simulink model "sim_pendulum"  (R2025b)
settings: Solver=FixedStepAuto  StartTime=0.0  StopTime=30  FixedStep=0.02  RelTol=1e-6
values from neighbouring files (symbols this model uses):
  c1 = m1*L_2 + m2 * LR    (= 0.0141005)    [sim_main.m]
  c2 = m1*L2_4 + m2 * LR2    (= 0.001480019375)    [sim_main.m]
  dx0 = 0    [KF_EKF_SIM_TEST.m]    (also in sim_main.m)
  g = 9.81    [sim_main.m]
  m1 = 0.0540    (= 0.054)    [sim_main.m]
  m2 = 0.0965    [sim_main.m]
  mu = 0.00015    [sim_main.m]
  x0 = [x0;dx0]    [KF_EKF_SIM_TEST.m]    (also in nss_pendulum_sim.m = zeros(2 + w_disturbance, 1); nss_pendulum_sim_dynamicchar.m = zeros(n, 1); nss_pendulum_sim_staticchar.m = zeros(n, 1); sim_main.m = deg2rad(45))
  xi = 0.0003    [sim_main.m]
libraries: simulink_extras x1
settings Model: Creator=rjrad  LastModifiedBy=rjrad
settings DataIOCC: SaveOutput=off  DSMLogging=off  SaveTime=off  ReturnWorkspaceOutputs=off

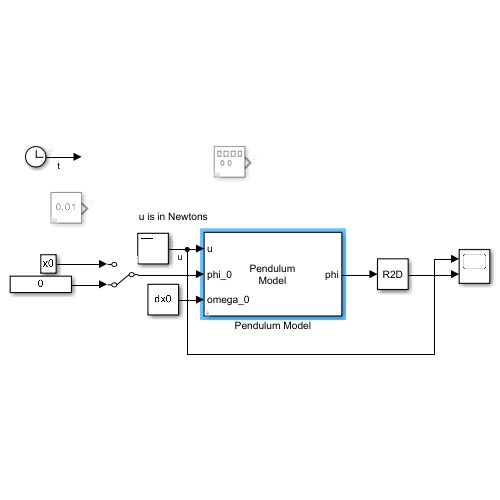
[thumbnail: Simulink's stored preview of the top-level diagram]
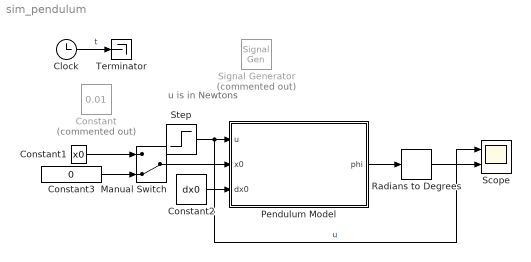
== system sim_pendulum ==
  note: u is in Newtons
  Clock : Clock
  Constant : Constant  Commented=on  Value=0.01
  Constant1 : Constant  Value=x0
  Constant2 : Constant  Value=dx0
  Constant3 : Constant  Value=0
  Manual Switch : ManualSwitch  CurrentSetting=0
  Pendulum Model : Subsystem  mask{g=g, b=xi, c1=c1, c2=c2}
      mask prompts: g "Gravitational acceleration"; b "Damping coefficient"; c1 "Inertia 1"; c2 "Inertia 2"
      mask Display:
      | disp('Pendulum\nModel');
      | port_label('output', 1, 'phi');
      | port_label('input', 1, 'u');
      | port_label('input', 2, 'phi_0');
      | port_label('input', 3, 'omega_0');
  Radians to Degrees : simulink_extras/Transformations/Radians to Degrees
  Scope : Scope  NumInputPorts=2
      settings: ActiveDisplayYMinimum=-15.510014538486551  ActiveDisplayYMaximum=16.134066660583571
  Signal Generator : SignalGenerator  Commented=on  WaveForm=sawtooth  Frequency=0.1
  Step : Step  Time=0.02  Before=0.15  After=0  SampleTime=0
  Terminator : Terminator
  wires:
  Radians to Degrees/1 -> Scope/2
  Clock/1 -> Terminator/1  "t"
  Step/1 -> Scope/1, Pendulum Model/1(u)  "u"
  Pendulum Model/1(phi) -> Radians to Degrees/1
  Constant3/1 -> Manual Switch/2
  Constant1/1 -> Manual Switch/1
  Constant2/1 -> Pendulum Model/3(dx0)
  Manual Switch/1 -> Pendulum Model/2(x0)

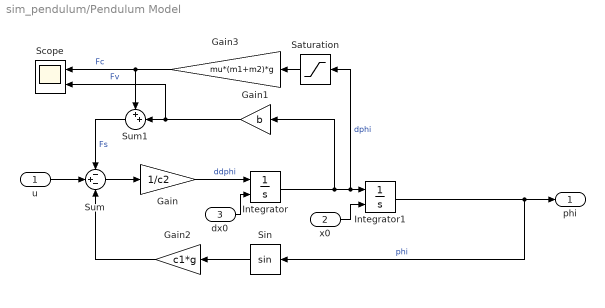
== system sim_pendulum/Pendulum Model ==
  u : Inport
  x0 : Inport  Port=2
  dx0 : Inport  Port=3
  Gain : Gain  Gain=1/c2
  Gain1 : Gain  Gain=b
  Gain2 : Gain  Gain=c1*g
  Gain3 : Gain  Gain=mu*(m1+m2)*g
  Integrator : Integrator  InitialConditionSource=external
  Integrator1 : Integrator  InitialConditionSource=external
  Saturation : Saturate  UpperLimit=1  LowerLimit=-1
  Scope : Scope  NumInputPorts=2
      settings: ActiveDisplayYMinimum=-0.00014295497944950421  ActiveDisplayYMaximum=6.11307568275033E-5
  Sin : Trigonometry
  Sum : Sum  Inputs=-+-
  Sum1 : Sum  Inputs=++|
  phi : Outport
  wires:
  Integrator1/1 -> phi/1, Sin/1  "phi"
  Gain/1 -> Integrator/1  "ddphi"
  Sin/1 -> Gain2/1
  Integrator/1 -> Gain1/1, Saturation/1, Integrator1/1  "dphi"
  Gain2/1 -> Sum/3
  Sum/1 -> Gain/1
  Gain1/1 -> Scope/2, Sum1/2  "Fv"
  dx0/1 -> Integrator/2
  x0/1 -> Integrator1/2
  u/1 -> Sum/2
  Saturation/1 -> Gain3/1
  Gain3/1 -> Scope/1, Sum1/1  "Fc"
  Sum1/1 -> Sum/1  "Fs"
